simulink model "Squelette_DSPB_ModulateurOQPSK"  (R2016a)
settings: Solver=FixedStepDiscrete  StartTime=0.0  StopTime=1e-3  RelTol=1e-3
InitFcn:
  | %% DSPBuilder Start
  | alt_dspbuilder_update_model(bdroot)
  | %% DSPBuilder End
libraries: allblocks_alteradspbuilder2 x243
(part 2 of 2)

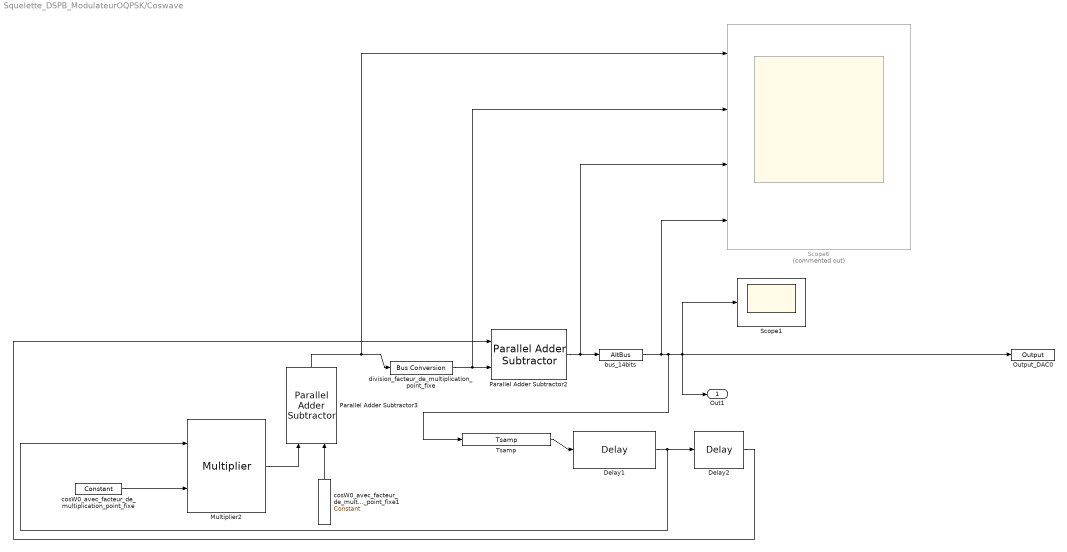
== system Squelette_DSPB_ModulateurOQPSK/Coswave ==
  Delay1 : allblocks_alteradspbuilder2/Delay  pipeline=1  pipeline_display=1  ClockPhase=1  use_ena=off  use_sclr=off  allowFloatingPointOverride=on  logOutputs=off  logFile=U:\S6\Projet\Squelette_ModulateurOQPSK__ORIG\tb_Squelette_DSPB_ModulateurOQPSK\Squelette%5FDSPB%5FModulateurOQPSK_Coswave_Delay1.fixedpointlog  use_init=on  reset_value=0.782390810576588
  Delay2 : allblocks_alteradspbuilder2/Delay  pipeline=1  pipeline_display=1  ClockPhase=1  use_ena=off  use_sclr=off  allowFloatingPointOverride=on  logOutputs=off  logFile=U:\S6\Projet\Squelette_ModulateurOQPSK__ORIG\tb_Squelette_DSPB_ModulateurOQPSK\Squelette%5FDSPB%5FModulateurOQPSK_Coswave_Delay2.fixedpointlog  use_init=on  reset_value=0.224270760949381
  Multiplier2 : allblocks_alteradspbuilder2/Multiplier  BusType=Signed Fractional  bwl=8  bwr=20  pipeline=0  pipeline_display=0  allowFloatingPointOverride=on  logOutputs=off  logFile=U:\S6\Projet\Squelette_ModulateurOQPSK__ORIG\tb_Squelette_DSPB_ModulateurOQPSK\Squelette%5FDSPB%5FModulateurOQPSK_Coswave_Multiplier2.fixedpointlog  UseEqualInputWidth=off  bbwl=8  bbwr=20  FullResolution=on  OutputMsb=8  OutputLsb=0  OutputBwl=16  OutputBwr=16  UseDedicatedCircuitry=YES  use_ena=off  use_aclr=off
  Output_DAC0 : allblocks_alteradspbuilder2/Output  iofile=U:\S6\Projet\Squelette_ModulateurOQPSK__ORIG\tb_Squelette_DSPB_ModulateurOQPSK\Squelette%5FDSPB%5FModulateurOQPSK_Coswave_Output%5FDAC0.capture  BusType=Signed Integer  bwl=14  bwr=0  externalType=Inferred  PORTTYPE=Output  allowFloatingPointOverride=on  logOutputs=off
  Parallel Adder Subtractor2 : allblocks_alteradspbuilder2/Parallel Adder Subtractor  number_of_inputs=2  direction=-+  use_pipeline=off  pipeline_display=0  phase_selection=1  use_ena=off  use_aclr=off  allowFloatingPointOverride=on  logOutputs=off  logFile=U:\S6\Projet\Squelette_ModulateurOQPSK__ORIG\tb_Squelette_DSPB_ModulateurOQPSK\Squelette%5FDSPB%5FModulateurOQPSK_Coswave_Parallel+Adder+Subtractor2.fixedpointlog
  Parallel Adder Subtractor3 : allblocks_alteradspbuilder2/Parallel Adder Subtractor  number_of_inputs=2  direction=+  use_pipeline=off  pipeline_display=0  phase_selection=1  use_ena=off  use_aclr=off  allowFloatingPointOverride=on  logOutputs=off  logFile=U:\S6\Projet\Squelette_ModulateurOQPSK__ORIG\tb_Squelette_DSPB_ModulateurOQPSK\Squelette%5FDSPB%5FModulateurOQPSK_Coswave_Parallel+Adder+Subtractor3.fixedpointlog
  Scope1 : Scope
  Scope6 : Scope  Commented=on  NumInputPorts=4
  Tsamp : allblocks_alteradspbuilder2/Tsamp  SpecifyClock=on  clock=Clock_100MHz
  bus_14bits : allblocks_alteradspbuilder2/AltBus  BusType=Signed Fractional  bwl=14  bwr=14  saturate=off  floatingPointInput=on  floatingPointOutput=on  logOutputs=off  logFile=U:\S6\Projet\Squelette_ModulateurOQPSK__ORIG\tb_Squelette_DSPB_ModulateurOQPSK\Squelette%5FDSPB%5FModulateurOQPSK_Coswave_bus%5F14bits.fixedpointlog
  cosW0_avec_facteur_de_multiplication_point_fixe : allblocks_alteradspbuilder2/Constant  mask_cst=1.564781621153176  BusType=Signed Fractional  bwl=19  bwr=19  roundMode=Truncate  satMode=Wrap  SpecifyClock=off  allowFloatingPointOverride=on  logOutputs=off  logFile=U:\S6\Projet\Squelette_ModulateurOQPSK__ORIG\tb_Squelette_DSPB_ModulateurOQPSK\Squelette%5FDSPB%5FModulateurOQPSK_Coswave_cosW0%5Favec%5Ffacteur%5Fde%5Fmultiplication%5Fpoint%5Ffixe.fixedpointlog
  cosW0_avec_facteur_de_multiplication_point_fixe1 : allblocks_alteradspbuilder2/Constant  mask_cst=2^-15  BusType=Signed Fractional  bwl=8  bwr=40  roundMode=Truncate  satMode=Wrap  SpecifyClock=off  allowFloatingPointOverride=on  logOutputs=off  logFile=U:\S6\Projet\Squelette_ModulateurOQPSK__ORIG\tb_Squelette_DSPB_ModulateurOQPSK\Squelette%5FDSPB%5FModulateurOQPSK_Coswave_cosW0%5Favec%5Ffacteur%5Fde%5Fmultiplication%5Fpoint%5Ffixe1.fixedpointlog
  division_facteur_de_multiplication_point_fixe : allblocks_alteradspbuilder2/Bus Conversion  BusType=Signed Fractional  ibwl=16  ibwr=40  bwl=8  bwr=20  bitToConnectToOutputLSB=16  round=off  saturate=off  pipeline_display=0
  Out1 : Outport
  wires:
  Parallel Adder Subtractor2/1 -> Scope6/3, bus_14bits/1
  Tsamp/1 -> Delay1/1
  cosW0_avec_facteur_de_multiplication_point_fixe1/1 -> Parallel Adder Subtractor3/2
  Multiplier2/1 -> Parallel Adder Subtractor3/1
  division_facteur_de_multiplication_point_fixe/1 -> Scope6/2, Parallel Adder Subtractor2/2
  Delay2/1 -> Parallel Adder Subtractor2/1
  Parallel Adder Subtractor3/1 -> Scope6/1, division_facteur_de_multiplication_point_fixe/1
  Delay1/1 -> Delay2/1, Multiplier2/1
  cosW0_avec_facteur_de_multiplication_point_fixe/1 -> Multiplier2/2
  bus_14bits/1 -> Scope6/4, Out1/1, Scope1/1, Output_DAC0/1, Tsamp/1

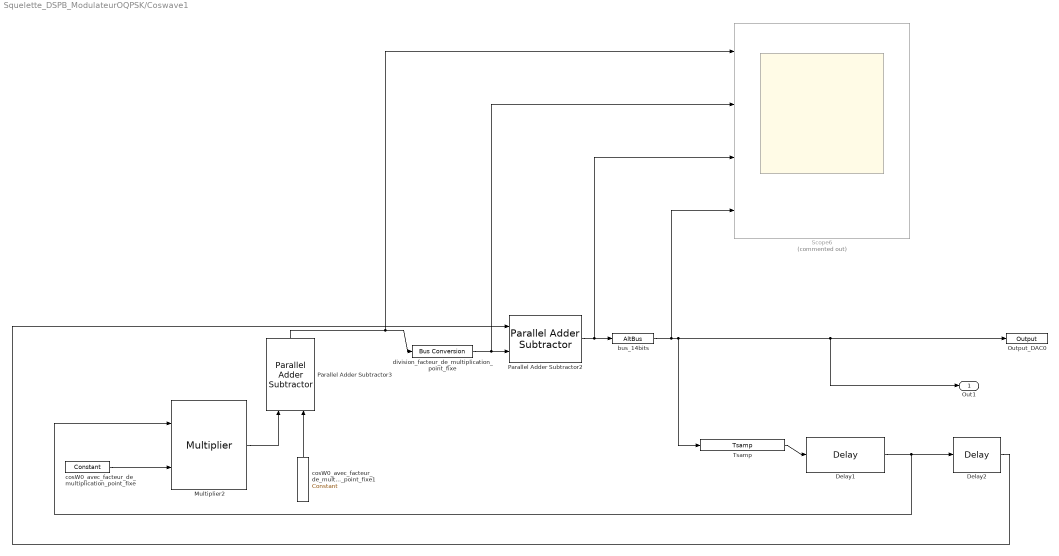
== system Squelette_DSPB_ModulateurOQPSK/Coswave1 ==
  Delay1 : allblocks_alteradspbuilder2/Delay  pipeline=1  pipeline_display=1  ClockPhase=1  use_ena=off  use_sclr=off  allowFloatingPointOverride=on  logOutputs=off  logFile=U:\S6\Projet\Squelette_ModulateurOQPSK__ORIG\tb_Squelette_DSPB_ModulateurOQPSK\Squelette%5FDSPB%5FModulateurOQPSK_Coswave1_Delay1.fixedpointlog  use_init=on  reset_value=0.782390810576588
  Delay2 : allblocks_alteradspbuilder2/Delay  pipeline=1  pipeline_display=1  ClockPhase=1  use_ena=off  use_sclr=off  allowFloatingPointOverride=on  logOutputs=off  logFile=U:\S6\Projet\Squelette_ModulateurOQPSK__ORIG\tb_Squelette_DSPB_ModulateurOQPSK\Squelette%5FDSPB%5FModulateurOQPSK_Coswave1_Delay2.fixedpointlog  use_init=on  reset_value=0.224270760949381
  Multiplier2 : allblocks_alteradspbuilder2/Multiplier  BusType=Signed Fractional  bwl=8  bwr=20  pipeline=0  pipeline_display=0  allowFloatingPointOverride=on  logOutputs=off  logFile=U:\S6\Projet\Squelette_ModulateurOQPSK__ORIG\tb_Squelette_DSPB_ModulateurOQPSK\Squelette%5FDSPB%5FModulateurOQPSK_Coswave1_Multiplier2.fixedpointlog  UseEqualInputWidth=off  bbwl=8  bbwr=20  FullResolution=on  OutputMsb=8  OutputLsb=0  OutputBwl=16  OutputBwr=16  UseDedicatedCircuitry=YES  use_ena=off  use_aclr=off
  Output_DAC0 : allblocks_alteradspbuilder2/Output  iofile=U:\S6\Projet\Squelette_ModulateurOQPSK__ORIG\tb_Squelette_DSPB_ModulateurOQPSK\Squelette%5FDSPB%5FModulateurOQPSK_Coswave1_Output%5FDAC0.capture  BusType=Signed Integer  bwl=14  bwr=0  externalType=Inferred  PORTTYPE=Output  allowFloatingPointOverride=on  logOutputs=off
  Parallel Adder Subtractor2 : allblocks_alteradspbuilder2/Parallel Adder Subtractor  number_of_inputs=2  direction=-+  use_pipeline=off  pipeline_display=0  phase_selection=1  use_ena=off  use_aclr=off  allowFloatingPointOverride=on  logOutputs=off  logFile=U:\S6\Projet\Squelette_ModulateurOQPSK__ORIG\tb_Squelette_DSPB_ModulateurOQPSK\Squelette%5FDSPB%5FModulateurOQPSK_Coswave1_Parallel+Adder+Subtractor2.fixedpointlog
  Parallel Adder Subtractor3 : allblocks_alteradspbuilder2/Parallel Adder Subtractor  number_of_inputs=2  direction=+  use_pipeline=off  pipeline_display=0  phase_selection=1  use_ena=off  use_aclr=off  allowFloatingPointOverride=on  logOutputs=off  logFile=U:\S6\Projet\Squelette_ModulateurOQPSK__ORIG\tb_Squelette_DSPB_ModulateurOQPSK\Squelette%5FDSPB%5FModulateurOQPSK_Coswave1_Parallel+Adder+Subtractor3.fixedpointlog
  Scope6 : Scope  Commented=on  NumInputPorts=4
  Tsamp : allblocks_alteradspbuilder2/Tsamp  SpecifyClock=on  clock=Clock_100MHz
  bus_14bits : allblocks_alteradspbuilder2/AltBus  BusType=Signed Fractional  bwl=14  bwr=14  saturate=off  floatingPointInput=on  floatingPointOutput=on  logOutputs=off  logFile=U:\S6\Projet\Squelette_ModulateurOQPSK__ORIG\tb_Squelette_DSPB_ModulateurOQPSK\Squelette%5FDSPB%5FModulateurOQPSK_Coswave1_bus%5F14bits.fixedpointlog
  cosW0_avec_facteur_de_multiplication_point_fixe : allblocks_alteradspbuilder2/Constant  mask_cst=1.564781621153176  BusType=Signed Fractional  bwl=19  bwr=19  roundMode=Truncate  satMode=Wrap  SpecifyClock=off  allowFloatingPointOverride=on  logOutputs=off  logFile=U:\S6\Projet\Squelette_ModulateurOQPSK__ORIG\tb_Squelette_DSPB_ModulateurOQPSK\Squelette%5FDSPB%5FModulateurOQPSK_Coswave1_cosW0%5Favec%5Ffacteur%5Fde%5Fmultiplication%5Fpoint%5Ffixe.fixedpointlog
  cosW0_avec_facteur_de_multiplication_point_fixe1 : allblocks_alteradspbuilder2/Constant  mask_cst=2^-15  BusType=Signed Fractional  bwl=8  bwr=40  roundMode=Truncate  satMode=Wrap  SpecifyClock=off  allowFloatingPointOverride=on  logOutputs=off  logFile=U:\S6\Projet\Squelette_ModulateurOQPSK__ORIG\tb_Squelette_DSPB_ModulateurOQPSK\Squelette%5FDSPB%5FModulateurOQPSK_Coswave1_cosW0%5Favec%5Ffacteur%5Fde%5Fmultiplication%5Fpoint%5Ffixe1.fixedpointlog
  division_facteur_de_multiplication_point_fixe : allblocks_alteradspbuilder2/Bus Conversion  BusType=Signed Fractional  ibwl=16  ibwr=40  bwl=8  bwr=20  bitToConnectToOutputLSB=16  round=off  saturate=off  pipeline_display=0
  Out1 : Outport
  wires:
  Parallel Adder Subtractor2/1 -> Scope6/3, bus_14bits/1
  Tsamp/1 -> Delay1/1
  cosW0_avec_facteur_de_multiplication_point_fixe1/1 -> Parallel Adder Subtractor3/2
  Multiplier2/1 -> Parallel Adder Subtractor3/1
  division_facteur_de_multiplication_point_fixe/1 -> Scope6/2, Parallel Adder Subtractor2/2
  Delay2/1 -> Parallel Adder Subtractor2/1
  Parallel Adder Subtractor3/1 -> Scope6/1, division_facteur_de_multiplication_point_fixe/1
  Delay1/1 -> Multiplier2/1, Delay2/1
  cosW0_avec_facteur_de_multiplication_point_fixe/1 -> Multiplier2/2
  bus_14bits/1 -> Scope6/4, Out1/1, Output_DAC0/1, Tsamp/1

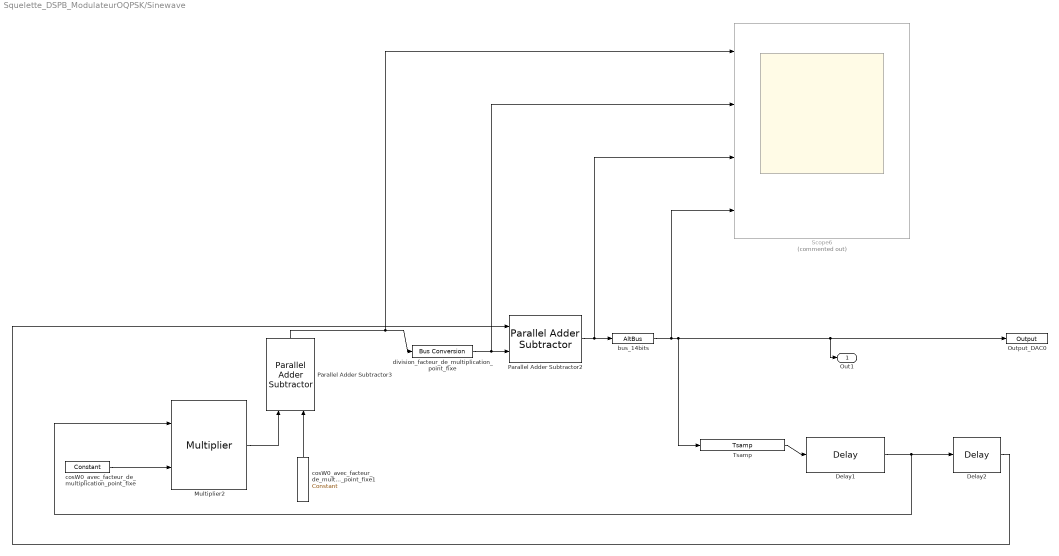
== system Squelette_DSPB_ModulateurOQPSK/Sinewave ==
  Delay1 : allblocks_alteradspbuilder2/Delay  pipeline=1  pipeline_display=1  ClockPhase=1  use_ena=off  use_sclr=off  allowFloatingPointOverride=on  logOutputs=off  logFile=U:\S6\Projet\Squelette_ModulateurOQPSK__ORIG\tb_Squelette_DSPB_ModulateurOQPSK\Squelette%5FDSPB%5FModulateurOQPSK_Sinewave_Delay1.fixedpointlog  use_init=on  reset_value=0.622787780488113
  Delay2 : allblocks_alteradspbuilder2/Delay  pipeline=1  pipeline_display=1  ClockPhase=1  use_ena=off  use_sclr=off  allowFloatingPointOverride=on  logOutputs=off  logFile=U:\S6\Projet\Squelette_ModulateurOQPSK__ORIG\tb_Squelette_DSPB_ModulateurOQPSK\Squelette%5FDSPB%5FModulateurOQPSK_Sinewave_Delay2.fixedpointlog  use_init=on  reset_value=0.974526872786577
  Multiplier2 : allblocks_alteradspbuilder2/Multiplier  BusType=Signed Fractional  bwl=8  bwr=20  pipeline=0  pipeline_display=0  allowFloatingPointOverride=on  logOutputs=off  logFile=U:\S6\Projet\Squelette_ModulateurOQPSK__ORIG\tb_Squelette_DSPB_ModulateurOQPSK\Squelette%5FDSPB%5FModulateurOQPSK_Sinewave_Multiplier2.fixedpointlog  UseEqualInputWidth=off  bbwl=8  bbwr=20  FullResolution=on  OutputMsb=8  OutputLsb=0  OutputBwl=16  OutputBwr=16  UseDedicatedCircuitry=YES  use_ena=off  use_aclr=off
  Output_DAC0 : allblocks_alteradspbuilder2/Output  iofile=U:\S6\Projet\Squelette_ModulateurOQPSK__ORIG\tb_Squelette_DSPB_ModulateurOQPSK\Squelette%5FDSPB%5FModulateurOQPSK_Sinewave_Output%5FDAC0.capture  BusType=Signed Integer  bwl=14  bwr=0  externalType=Inferred  PORTTYPE=Output  allowFloatingPointOverride=on  logOutputs=off
  Parallel Adder Subtractor2 : allblocks_alteradspbuilder2/Parallel Adder Subtractor  number_of_inputs=2  direction=-+  use_pipeline=off  pipeline_display=0  phase_selection=1  use_ena=off  use_aclr=off  allowFloatingPointOverride=on  logOutputs=off  logFile=U:\S6\Projet\Squelette_ModulateurOQPSK__ORIG\tb_Squelette_DSPB_ModulateurOQPSK\Squelette%5FDSPB%5FModulateurOQPSK_Sinewave_Parallel+Adder+Subtractor2.fixedpointlog
  Parallel Adder Subtractor3 : allblocks_alteradspbuilder2/Parallel Adder Subtractor  number_of_inputs=2  direction=+  use_pipeline=off  pipeline_display=0  phase_selection=1  use_ena=off  use_aclr=off  allowFloatingPointOverride=on  logOutputs=off  logFile=U:\S6\Projet\Squelette_ModulateurOQPSK__ORIG\tb_Squelette_DSPB_ModulateurOQPSK\Squelette%5FDSPB%5FModulateurOQPSK_Sinewave_Parallel+Adder+Subtractor3.fixedpointlog
  Scope6 : Scope  Commented=on  NumInputPorts=4
  Tsamp : allblocks_alteradspbuilder2/Tsamp  SpecifyClock=on  clock=Clock_100MHz
  bus_14bits : allblocks_alteradspbuilder2/AltBus  BusType=Signed Fractional  bwl=14  bwr=14  saturate=off  floatingPointInput=on  floatingPointOutput=on  logOutputs=off  logFile=U:\S6\Projet\Squelette_ModulateurOQPSK__ORIG\tb_Squelette_DSPB_ModulateurOQPSK\Squelette%5FDSPB%5FModulateurOQPSK_Sinewave_bus%5F14bits.fixedpointlog
  cosW0_avec_facteur_de_multiplication_point_fixe : allblocks_alteradspbuilder2/Constant  mask_cst=1.564781621153176  BusType=Signed Fractional  bwl=19  bwr=19  roundMode=Truncate  satMode=Wrap  SpecifyClock=off  allowFloatingPointOverride=on  logOutputs=off  logFile=U:\S6\Projet\Squelette_ModulateurOQPSK__ORIG\tb_Squelette_DSPB_ModulateurOQPSK\Squelette%5FDSPB%5FModulateurOQPSK_Sinewave_cosW0%5Favec%5Ffacteur%5Fde%5Fmultiplication%5Fpoint%5Ffixe.fixedpointlog
  cosW0_avec_facteur_de_multiplication_point_fixe1 : allblocks_alteradspbuilder2/Constant  mask_cst=2^-15  BusType=Signed Fractional  bwl=8  bwr=40  roundMode=Truncate  satMode=Wrap  SpecifyClock=off  allowFloatingPointOverride=on  logOutputs=off  logFile=U:\S6\Projet\Squelette_ModulateurOQPSK__ORIG\tb_Squelette_DSPB_ModulateurOQPSK\Squelette%5FDSPB%5FModulateurOQPSK_Sinewave_cosW0%5Favec%5Ffacteur%5Fde%5Fmultiplication%5Fpoint%5Ffixe1.fixedpointlog
  division_facteur_de_multiplication_point_fixe : allblocks_alteradspbuilder2/Bus Conversion  BusType=Signed Fractional  ibwl=16  ibwr=40  bwl=8  bwr=20  bitToConnectToOutputLSB=16  round=off  saturate=off  pipeline_display=0
  Out1 : Outport
  wires:
  Parallel Adder Subtractor2/1 -> Scope6/3, bus_14bits/1
  Tsamp/1 -> Delay1/1
  cosW0_avec_facteur_de_multiplication_point_fixe1/1 -> Parallel Adder Subtractor3/2
  Multiplier2/1 -> Parallel Adder Subtractor3/1
  division_facteur_de_multiplication_point_fixe/1 -> Scope6/2, Parallel Adder Subtractor2/2
  Delay2/1 -> Parallel Adder Subtractor2/1
  Parallel Adder Subtractor3/1 -> Scope6/1, division_facteur_de_multiplication_point_fixe/1
  Delay1/1 -> Multiplier2/1, Delay2/1
  cosW0_avec_facteur_de_multiplication_point_fixe/1 -> Multiplier2/2
  bus_14bits/1 -> Scope6/4, Out1/1, Output_DAC0/1, Tsamp/1

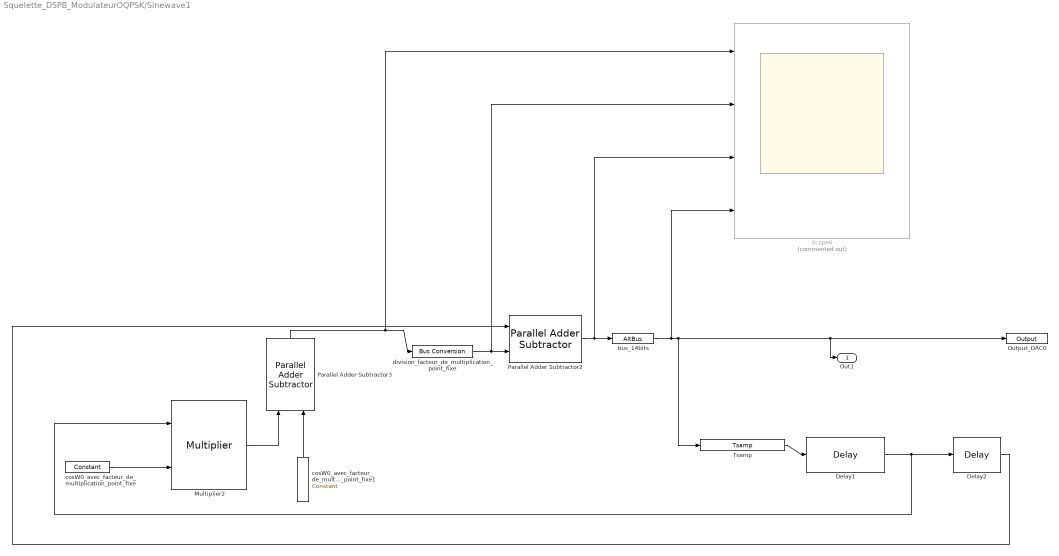
== system Squelette_DSPB_ModulateurOQPSK/Sinewave1 ==
  Delay1 : allblocks_alteradspbuilder2/Delay  pipeline=1  pipeline_display=1  ClockPhase=1  use_ena=off  use_sclr=off  allowFloatingPointOverride=on  logOutputs=off  logFile=U:\S6\Projet\Squelette_ModulateurOQPSK__ORIG\tb_Squelette_DSPB_ModulateurOQPSK\Squelette%5FDSPB%5FModulateurOQPSK_Sinewave1_Delay1.fixedpointlog  use_init=on  reset_value=0.031410759078128
  Delay2 : allblocks_alteradspbuilder2/Delay  pipeline=1  pipeline_display=1  ClockPhase=1  use_ena=off  use_sclr=off  allowFloatingPointOverride=on  logOutputs=off  logFile=U:\S6\Projet\Squelette_ModulateurOQPSK__ORIG\tb_Squelette_DSPB_ModulateurOQPSK\Squelette%5FDSPB%5FModulateurOQPSK_Sinewave1_Delay2.fixedpointlog  use_init=on  reset_value=0.062790519529314
  Multiplier2 : allblocks_alteradspbuilder2/Multiplier  BusType=Signed Fractional  bwl=8  bwr=20  pipeline=0  pipeline_display=0  allowFloatingPointOverride=on  logOutputs=off  logFile=U:\S6\Projet\Squelette_ModulateurOQPSK__ORIG\tb_Squelette_DSPB_ModulateurOQPSK\Squelette%5FDSPB%5FModulateurOQPSK_Sinewave1_Multiplier2.fixedpointlog  UseEqualInputWidth=off  bbwl=8  bbwr=20  FullResolution=on  OutputMsb=8  OutputLsb=0  OutputBwl=16  OutputBwr=16  UseDedicatedCircuitry=YES  use_ena=off  use_aclr=off
  Output_DAC0 : allblocks_alteradspbuilder2/Output  iofile=U:\S6\Projet\Squelette_ModulateurOQPSK__ORIG\tb_Squelette_DSPB_ModulateurOQPSK\Squelette%5FDSPB%5FModulateurOQPSK_Sinewave1_Output%5FDAC0.capture  BusType=Signed Integer  bwl=14  bwr=0  externalType=Inferred  PORTTYPE=Output  allowFloatingPointOverride=on  logOutputs=off
  Parallel Adder Subtractor2 : allblocks_alteradspbuilder2/Parallel Adder Subtractor  number_of_inputs=2  direction=-+  use_pipeline=off  pipeline_display=0  phase_selection=1  use_ena=off  use_aclr=off  allowFloatingPointOverride=on  logOutputs=off  logFile=U:\S6\Projet\Squelette_ModulateurOQPSK__ORIG\tb_Squelette_DSPB_ModulateurOQPSK\Squelette%5FDSPB%5FModulateurOQPSK_Sinewave1_Parallel+Adder+Subtractor2.fixedpointlog
  Parallel Adder Subtractor3 : allblocks_alteradspbuilder2/Parallel Adder Subtractor  number_of_inputs=2  direction=+  use_pipeline=off  pipeline_display=0  phase_selection=1  use_ena=off  use_aclr=off  allowFloatingPointOverride=on  logOutputs=off  logFile=U:\S6\Projet\Squelette_ModulateurOQPSK__ORIG\tb_Squelette_DSPB_ModulateurOQPSK\Squelette%5FDSPB%5FModulateurOQPSK_Sinewave1_Parallel+Adder+Subtractor3.fixedpointlog
  Scope6 : Scope  Commented=on  NumInputPorts=4
  Tsamp : allblocks_alteradspbuilder2/Tsamp  SpecifyClock=on  clock=Clock_100MHz
  bus_14bits : allblocks_alteradspbuilder2/AltBus  BusType=Signed Fractional  bwl=14  bwr=14  saturate=off  floatingPointInput=on  floatingPointOutput=on  logOutputs=off  logFile=U:\S6\Projet\Squelette_ModulateurOQPSK__ORIG\tb_Squelette_DSPB_ModulateurOQPSK\Squelette%5FDSPB%5FModulateurOQPSK_Sinewave1_bus%5F14bits.fixedpointlog
  cosW0_avec_facteur_de_multiplication_point_fixe : allblocks_alteradspbuilder2/Constant  mask_cst=1.999013120731463  BusType=Signed Fractional  bwl=19  bwr=19  roundMode=Truncate  satMode=Wrap  SpecifyClock=off  allowFloatingPointOverride=on  logOutputs=off  logFile=U:\S6\Projet\Squelette_ModulateurOQPSK__ORIG\tb_Squelette_DSPB_ModulateurOQPSK\Squelette%5FDSPB%5FModulateurOQPSK_Sinewave1_cosW0%5Favec%5Ffacteur%5Fde%5Fmultiplication%5Fpoint%5Ffixe.fixedpointlog
  cosW0_avec_facteur_de_multiplication_point_fixe1 : allblocks_alteradspbuilder2/Constant  mask_cst=2^-15  BusType=Signed Fractional  bwl=8  bwr=40  roundMode=Truncate  satMode=Wrap  SpecifyClock=off  allowFloatingPointOverride=on  logOutputs=off  logFile=U:\S6\Projet\Squelette_ModulateurOQPSK__ORIG\tb_Squelette_DSPB_ModulateurOQPSK\Squelette%5FDSPB%5FModulateurOQPSK_Sinewave1_cosW0%5Favec%5Ffacteur%5Fde%5Fmultiplication%5Fpoint%5Ffixe1.fixedpointlog
  division_facteur_de_multiplication_point_fixe : allblocks_alteradspbuilder2/Bus Conversion  BusType=Signed Fractional  ibwl=16  ibwr=40  bwl=8  bwr=20  bitToConnectToOutputLSB=16  round=off  saturate=off  pipeline_display=0
  Out1 : Outport
  wires:
  Parallel Adder Subtractor2/1 -> Scope6/3, bus_14bits/1
  Tsamp/1 -> Delay1/1
  cosW0_avec_facteur_de_multiplication_point_fixe1/1 -> Parallel Adder Subtractor3/2
  Multiplier2/1 -> Parallel Adder Subtractor3/1
  division_facteur_de_multiplication_point_fixe/1 -> Scope6/2, Parallel Adder Subtractor2/2
  Delay2/1 -> Parallel Adder Subtractor2/1
  Parallel Adder Subtractor3/1 -> Scope6/1, division_facteur_de_multiplication_point_fixe/1
  Delay1/1 -> Multiplier2/1, Delay2/1
  cosW0_avec_facteur_de_multiplication_point_fixe/1 -> Multiplier2/2
  bus_14bits/1 -> Scope6/4, Out1/1, Output_DAC0/1, Tsamp/1

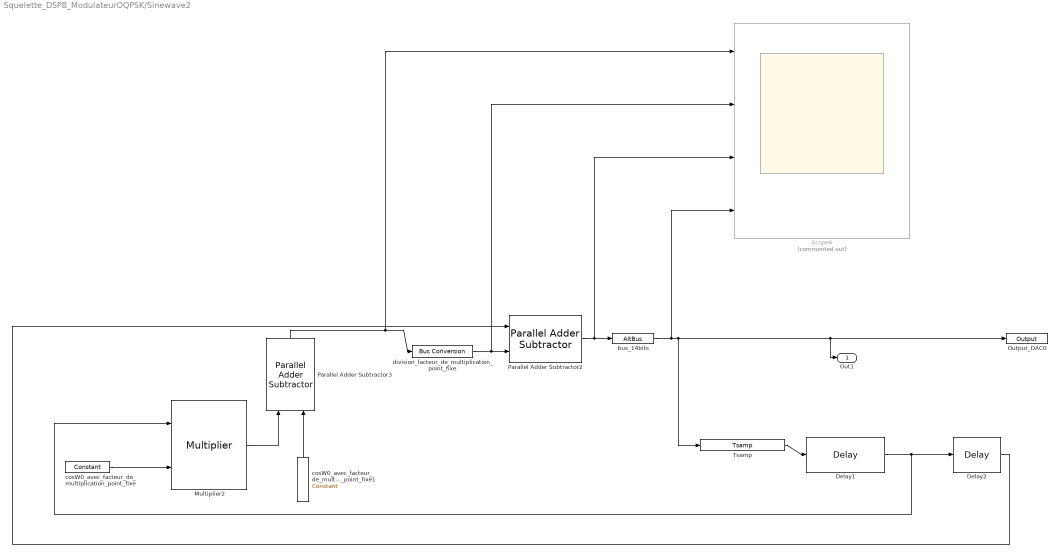
== system Squelette_DSPB_ModulateurOQPSK/Sinewave2 ==
  Delay1 : allblocks_alteradspbuilder2/Delay  pipeline=1  pipeline_display=1  ClockPhase=1  use_ena=off  use_sclr=off  allowFloatingPointOverride=on  logOutputs=off  logFile=U:\S6\Projet\Squelette_ModulateurOQPSK__ORIG\tb_Squelette_DSPB_ModulateurOQPSK\Squelette%5FDSPB%5FModulateurOQPSK_Sinewave2_Delay1.fixedpointlog  use_init=on  reset_value=0.031410759078128
  Delay2 : allblocks_alteradspbuilder2/Delay  pipeline=1  pipeline_display=1  ClockPhase=1  use_ena=off  use_sclr=off  allowFloatingPointOverride=on  logOutputs=off  logFile=U:\S6\Projet\Squelette_ModulateurOQPSK__ORIG\tb_Squelette_DSPB_ModulateurOQPSK\Squelette%5FDSPB%5FModulateurOQPSK_Sinewave2_Delay2.fixedpointlog  use_init=on  reset_value=0.062790519529314
  Multiplier2 : allblocks_alteradspbuilder2/Multiplier  BusType=Signed Fractional  bwl=8  bwr=20  pipeline=0  pipeline_display=0  allowFloatingPointOverride=on  logOutputs=off  logFile=U:\S6\Projet\Squelette_ModulateurOQPSK__ORIG\tb_Squelette_DSPB_ModulateurOQPSK\Squelette%5FDSPB%5FModulateurOQPSK_Sinewave2_Multiplier2.fixedpointlog  UseEqualInputWidth=off  bbwl=8  bbwr=20  FullResolution=on  OutputMsb=8  OutputLsb=0  OutputBwl=16  OutputBwr=16  UseDedicatedCircuitry=YES  use_ena=off  use_aclr=off
  Output_DAC0 : allblocks_alteradspbuilder2/Output  iofile=U:\S6\Projet\Squelette_ModulateurOQPSK__ORIG\tb_Squelette_DSPB_ModulateurOQPSK\Squelette%5FDSPB%5FModulateurOQPSK_Sinewave2_Output%5FDAC0.capture  BusType=Signed Integer  bwl=14  bwr=0  externalType=Inferred  PORTTYPE=Output  allowFloatingPointOverride=on  logOutputs=off
  Parallel Adder Subtractor2 : allblocks_alteradspbuilder2/Parallel Adder Subtractor  number_of_inputs=2  direction=-+  use_pipeline=off  pipeline_display=0  phase_selection=1  use_ena=off  use_aclr=off  allowFloatingPointOverride=on  logOutputs=off  logFile=U:\S6\Projet\Squelette_ModulateurOQPSK__ORIG\tb_Squelette_DSPB_ModulateurOQPSK\Squelette%5FDSPB%5FModulateurOQPSK_Sinewave2_Parallel+Adder+Subtractor2.fixedpointlog
  Parallel Adder Subtractor3 : allblocks_alteradspbuilder2/Parallel Adder Subtractor  number_of_inputs=2  direction=+  use_pipeline=off  pipeline_display=0  phase_selection=1  use_ena=off  use_aclr=off  allowFloatingPointOverride=on  logOutputs=off  logFile=U:\S6\Projet\Squelette_ModulateurOQPSK__ORIG\tb_Squelette_DSPB_ModulateurOQPSK\Squelette%5FDSPB%5FModulateurOQPSK_Sinewave2_Parallel+Adder+Subtractor3.fixedpointlog
  Scope6 : Scope  Commented=on  NumInputPorts=4
  Tsamp : allblocks_alteradspbuilder2/Tsamp  SpecifyClock=on  clock=Clock_100MHz
  bus_14bits : allblocks_alteradspbuilder2/AltBus  BusType=Signed Fractional  bwl=14  bwr=14  saturate=off  floatingPointInput=on  floatingPointOutput=on  logOutputs=off  logFile=U:\S6\Projet\Squelette_ModulateurOQPSK__ORIG\tb_Squelette_DSPB_ModulateurOQPSK\Squelette%5FDSPB%5FModulateurOQPSK_Sinewave2_bus%5F14bits.fixedpointlog
  cosW0_avec_facteur_de_multiplication_point_fixe : allblocks_alteradspbuilder2/Constant  mask_cst=1.999013120731463  BusType=Signed Fractional  bwl=19  bwr=19  roundMode=Truncate  satMode=Wrap  SpecifyClock=off  allowFloatingPointOverride=on  logOutputs=off  logFile=U:\S6\Projet\Squelette_ModulateurOQPSK__ORIG\tb_Squelette_DSPB_ModulateurOQPSK\Squelette%5FDSPB%5FModulateurOQPSK_Sinewave2_cosW0%5Favec%5Ffacteur%5Fde%5Fmultiplication%5Fpoint%5Ffixe.fixedpointlog
  cosW0_avec_facteur_de_multiplication_point_fixe1 : allblocks_alteradspbuilder2/Constant  mask_cst=2^-15  BusType=Signed Fractional  bwl=8  bwr=40  roundMode=Truncate  satMode=Wrap  SpecifyClock=off  allowFloatingPointOverride=on  logOutputs=off  logFile=U:\S6\Projet\Squelette_ModulateurOQPSK__ORIG\tb_Squelette_DSPB_ModulateurOQPSK\Squelette%5FDSPB%5FModulateurOQPSK_Sinewave2_cosW0%5Favec%5Ffacteur%5Fde%5Fmultiplication%5Fpoint%5Ffixe1.fixedpointlog
  division_facteur_de_multiplication_point_fixe : allblocks_alteradspbuilder2/Bus Conversion  BusType=Signed Fractional  ibwl=16  ibwr=40  bwl=8  bwr=20  bitToConnectToOutputLSB=16  round=off  saturate=off  pipeline_display=0
  Out1 : Outport
  wires:
  Parallel Adder Subtractor2/1 -> Scope6/3, bus_14bits/1
  Tsamp/1 -> Delay1/1
  cosW0_avec_facteur_de_multiplication_point_fixe1/1 -> Parallel Adder Subtractor3/2
  Multiplier2/1 -> Parallel Adder Subtractor3/1
  division_facteur_de_multiplication_point_fixe/1 -> Scope6/2, Parallel Adder Subtractor2/2
  Delay2/1 -> Parallel Adder Subtractor2/1
  Parallel Adder Subtractor3/1 -> Scope6/1, division_facteur_de_multiplication_point_fixe/1
  Delay1/1 -> Multiplier2/1, Delay2/1
  cosW0_avec_facteur_de_multiplication_point_fixe/1 -> Multiplier2/2
  bus_14bits/1 -> Scope6/4, Out1/1, Output_DAC0/1, Tsamp/1

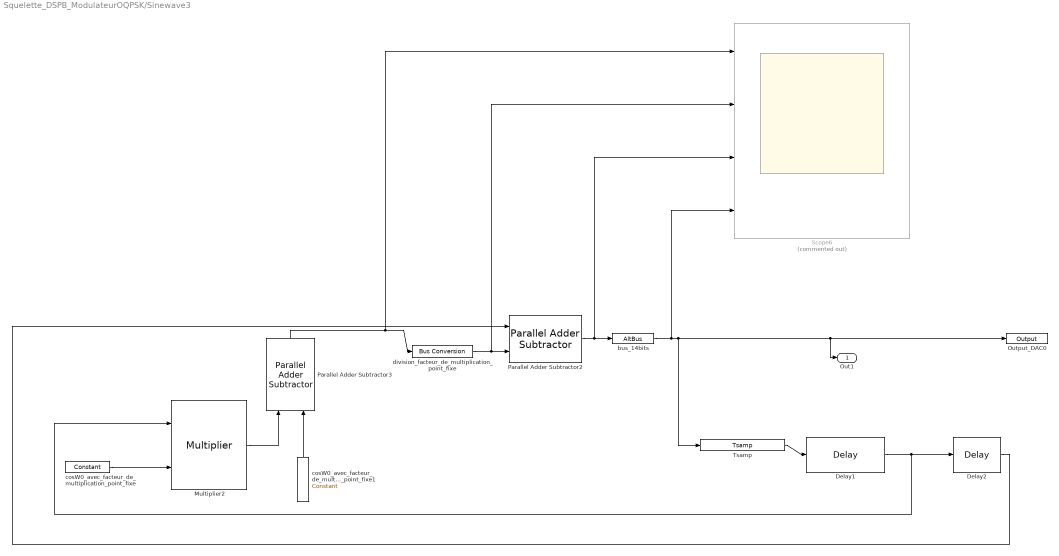
== system Squelette_DSPB_ModulateurOQPSK/Sinewave3 ==
  Delay1 : allblocks_alteradspbuilder2/Delay  pipeline=1  pipeline_display=1  ClockPhase=1  use_ena=off  use_sclr=off  allowFloatingPointOverride=on  logOutputs=off  logFile=U:\S6\Projet\Squelette_ModulateurOQPSK__ORIG\tb_Squelette_DSPB_ModulateurOQPSK\Squelette%5FDSPB%5FModulateurOQPSK_Sinewave3_Delay1.fixedpointlog  use_init=on  reset_value=0.622787780488113
  Delay2 : allblocks_alteradspbuilder2/Delay  pipeline=1  pipeline_display=1  ClockPhase=1  use_ena=off  use_sclr=off  allowFloatingPointOverride=on  logOutputs=off  logFile=U:\S6\Projet\Squelette_ModulateurOQPSK__ORIG\tb_Squelette_DSPB_ModulateurOQPSK\Squelette%5FDSPB%5FModulateurOQPSK_Sinewave3_Delay2.fixedpointlog  use_init=on  reset_value=0.974526872786577
  Multiplier2 : allblocks_alteradspbuilder2/Multiplier  BusType=Signed Fractional  bwl=8  bwr=20  pipeline=0  pipeline_display=0  allowFloatingPointOverride=on  logOutputs=off  logFile=U:\S6\Projet\Squelette_ModulateurOQPSK__ORIG\tb_Squelette_DSPB_ModulateurOQPSK\Squelette%5FDSPB%5FModulateurOQPSK_Sinewave3_Multiplier2.fixedpointlog  UseEqualInputWidth=off  bbwl=8  bbwr=20  FullResolution=on  OutputMsb=8  OutputLsb=0  OutputBwl=16  OutputBwr=16  UseDedicatedCircuitry=YES  use_ena=off  use_aclr=off
  Output_DAC0 : allblocks_alteradspbuilder2/Output  iofile=U:\S6\Projet\Squelette_ModulateurOQPSK__ORIG\tb_Squelette_DSPB_ModulateurOQPSK\Squelette%5FDSPB%5FModulateurOQPSK_Sinewave3_Output%5FDAC0.capture  BusType=Signed Integer  bwl=14  bwr=0  externalType=Inferred  PORTTYPE=Output  allowFloatingPointOverride=on  logOutputs=off
  Parallel Adder Subtractor2 : allblocks_alteradspbuilder2/Parallel Adder Subtractor  number_of_inputs=2  direction=-+  use_pipeline=off  pipeline_display=0  phase_selection=1  use_ena=off  use_aclr=off  allowFloatingPointOverride=on  logOutputs=off  logFile=U:\S6\Projet\Squelette_ModulateurOQPSK__ORIG\tb_Squelette_DSPB_ModulateurOQPSK\Squelette%5FDSPB%5FModulateurOQPSK_Sinewave3_Parallel+Adder+Subtractor2.fixedpointlog
  Parallel Adder Subtractor3 : allblocks_alteradspbuilder2/Parallel Adder Subtractor  number_of_inputs=2  direction=+  use_pipeline=off  pipeline_display=0  phase_selection=1  use_ena=off  use_aclr=off  allowFloatingPointOverride=on  logOutputs=off  logFile=U:\S6\Projet\Squelette_ModulateurOQPSK__ORIG\tb_Squelette_DSPB_ModulateurOQPSK\Squelette%5FDSPB%5FModulateurOQPSK_Sinewave3_Parallel+Adder+Subtractor3.fixedpointlog
  Scope6 : Scope  Commented=on  NumInputPorts=4
  Tsamp : allblocks_alteradspbuilder2/Tsamp  SpecifyClock=on  clock=Clock_100MHz
  bus_14bits : allblocks_alteradspbuilder2/AltBus  BusType=Signed Fractional  bwl=14  bwr=14  saturate=off  floatingPointInput=on  floatingPointOutput=on  logOutputs=off  logFile=U:\S6\Projet\Squelette_ModulateurOQPSK__ORIG\tb_Squelette_DSPB_ModulateurOQPSK\Squelette%5FDSPB%5FModulateurOQPSK_Sinewave3_bus%5F14bits.fixedpointlog
  cosW0_avec_facteur_de_multiplication_point_fixe : allblocks_alteradspbuilder2/Constant  mask_cst=1.564781621153176  BusType=Signed Fractional  bwl=19  bwr=19  roundMode=Truncate  satMode=Wrap  SpecifyClock=off  allowFloatingPointOverride=on  logOutputs=off  logFile=U:\S6\Projet\Squelette_ModulateurOQPSK__ORIG\tb_Squelette_DSPB_ModulateurOQPSK\Squelette%5FDSPB%5FModulateurOQPSK_Sinewave3_cosW0%5Favec%5Ffacteur%5Fde%5Fmultiplication%5Fpoint%5Ffixe.fixedpointlog
  cosW0_avec_facteur_de_multiplication_point_fixe1 : allblocks_alteradspbuilder2/Constant  mask_cst=2^-15  BusType=Signed Fractional  bwl=8  bwr=40  roundMode=Truncate  satMode=Wrap  SpecifyClock=off  allowFloatingPointOverride=on  logOutputs=off  logFile=U:\S6\Projet\Squelette_ModulateurOQPSK__ORIG\tb_Squelette_DSPB_ModulateurOQPSK\Squelette%5FDSPB%5FModulateurOQPSK_Sinewave3_cosW0%5Favec%5Ffacteur%5Fde%5Fmultiplication%5Fpoint%5Ffixe1.fixedpointlog
  division_facteur_de_multiplication_point_fixe : allblocks_alteradspbuilder2/Bus Conversion  BusType=Signed Fractional  ibwl=16  ibwr=40  bwl=8  bwr=20  bitToConnectToOutputLSB=16  round=off  saturate=off  pipeline_display=0
  Out1 : Outport
  wires:
  Parallel Adder Subtractor2/1 -> Scope6/3, bus_14bits/1
  Tsamp/1 -> Delay1/1
  cosW0_avec_facteur_de_multiplication_point_fixe1/1 -> Parallel Adder Subtractor3/2
  Multiplier2/1 -> Parallel Adder Subtractor3/1
  division_facteur_de_multiplication_point_fixe/1 -> Scope6/2, Parallel Adder Subtractor2/2
  Delay2/1 -> Parallel Adder Subtractor2/1
  Parallel Adder Subtractor3/1 -> Scope6/1, division_facteur_de_multiplication_point_fixe/1
  Delay1/1 -> Multiplier2/1, Delay2/1
  cosW0_avec_facteur_de_multiplication_point_fixe/1 -> Multiplier2/2
  bus_14bits/1 -> Scope6/4, Out1/1, Output_DAC0/1, Tsamp/1

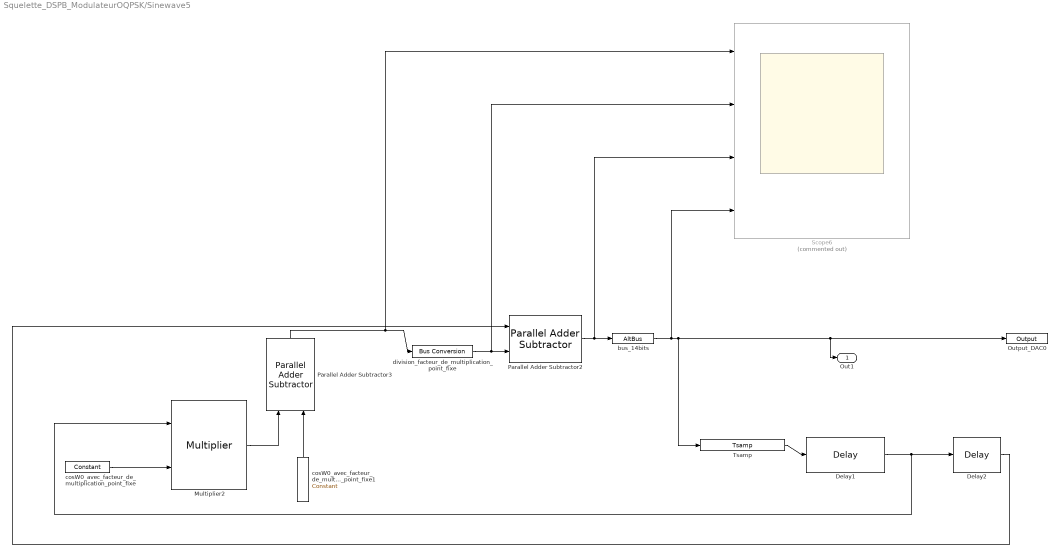
== system Squelette_DSPB_ModulateurOQPSK/Sinewave5 ==
  Delay1 : allblocks_alteradspbuilder2/Delay  pipeline=1  pipeline_display=1  ClockPhase=1  use_ena=off  use_sclr=off  allowFloatingPointOverride=on  logOutputs=off  logFile=U:\S6\Projet\Squelette_ModulateurOQPSK__ORIG\tb_Squelette_DSPB_ModulateurOQPSK\Squelette%5FDSPB%5FModulateurOQPSK_Sinewave5_Delay1.fixedpointlog  use_init=on  reset_value=0.031410759078128
  Delay2 : allblocks_alteradspbuilder2/Delay  pipeline=1  pipeline_display=1  ClockPhase=1  use_ena=off  use_sclr=off  allowFloatingPointOverride=on  logOutputs=off  logFile=U:\S6\Projet\Squelette_ModulateurOQPSK__ORIG\tb_Squelette_DSPB_ModulateurOQPSK\Squelette%5FDSPB%5FModulateurOQPSK_Sinewave5_Delay2.fixedpointlog  use_init=on  reset_value=0.062790519529314
  Multiplier2 : allblocks_alteradspbuilder2/Multiplier  BusType=Signed Fractional  bwl=8  bwr=20  pipeline=0  pipeline_display=0  allowFloatingPointOverride=on  logOutputs=off  logFile=U:\S6\Projet\Squelette_ModulateurOQPSK__ORIG\tb_Squelette_DSPB_ModulateurOQPSK\Squelette%5FDSPB%5FModulateurOQPSK_Sinewave5_Multiplier2.fixedpointlog  UseEqualInputWidth=off  bbwl=8  bbwr=20  FullResolution=on  OutputMsb=8  OutputLsb=0  OutputBwl=16  OutputBwr=16  UseDedicatedCircuitry=YES  use_ena=off  use_aclr=off
  Output_DAC0 : allblocks_alteradspbuilder2/Output  iofile=U:\S6\Projet\Squelette_ModulateurOQPSK__ORIG\tb_Squelette_DSPB_ModulateurOQPSK\Squelette%5FDSPB%5FModulateurOQPSK_Sinewave5_Output%5FDAC0.capture  BusType=Signed Integer  bwl=14  bwr=0  externalType=Inferred  PORTTYPE=Output  allowFloatingPointOverride=on  logOutputs=off
  Parallel Adder Subtractor2 : allblocks_alteradspbuilder2/Parallel Adder Subtractor  number_of_inputs=2  direction=-+  use_pipeline=off  pipeline_display=0  phase_selection=1  use_ena=off  use_aclr=off  allowFloatingPointOverride=on  logOutputs=off  logFile=U:\S6\Projet\Squelette_ModulateurOQPSK__ORIG\tb_Squelette_DSPB_ModulateurOQPSK\Squelette%5FDSPB%5FModulateurOQPSK_Sinewave5_Parallel+Adder+Subtractor2.fixedpointlog
  Parallel Adder Subtractor3 : allblocks_alteradspbuilder2/Parallel Adder Subtractor  number_of_inputs=2  direction=+  use_pipeline=off  pipeline_display=0  phase_selection=1  use_ena=off  use_aclr=off  allowFloatingPointOverride=on  logOutputs=off  logFile=U:\S6\Projet\Squelette_ModulateurOQPSK__ORIG\tb_Squelette_DSPB_ModulateurOQPSK\Squelette%5FDSPB%5FModulateurOQPSK_Sinewave5_Parallel+Adder+Subtractor3.fixedpointlog
  Scope6 : Scope  Commented=on  NumInputPorts=4
  Tsamp : allblocks_alteradspbuilder2/Tsamp  SpecifyClock=on  clock=Clock_100MHz
  bus_14bits : allblocks_alteradspbuilder2/AltBus  BusType=Signed Fractional  bwl=14  bwr=14  saturate=off  floatingPointInput=on  floatingPointOutput=on  logOutputs=off  logFile=U:\S6\Projet\Squelette_ModulateurOQPSK__ORIG\tb_Squelette_DSPB_ModulateurOQPSK\Squelette%5FDSPB%5FModulateurOQPSK_Sinewave5_bus%5F14bits.fixedpointlog
  cosW0_avec_facteur_de_multiplication_point_fixe : allblocks_alteradspbuilder2/Constant  mask_cst=1.999013120731463  BusType=Signed Fractional  bwl=19  bwr=19  roundMode=Truncate  satMode=Wrap  SpecifyClock=off  allowFloatingPointOverride=on  logOutputs=off  logFile=U:\S6\Projet\Squelette_ModulateurOQPSK__ORIG\tb_Squelette_DSPB_ModulateurOQPSK\Squelette%5FDSPB%5FModulateurOQPSK_Sinewave5_cosW0%5Favec%5Ffacteur%5Fde%5Fmultiplication%5Fpoint%5Ffixe.fixedpointlog
  cosW0_avec_facteur_de_multiplication_point_fixe1 : allblocks_alteradspbuilder2/Constant  mask_cst=2^-15  BusType=Signed Fractional  bwl=8  bwr=40  roundMode=Truncate  satMode=Wrap  SpecifyClock=off  allowFloatingPointOverride=on  logOutputs=off  logFile=U:\S6\Projet\Squelette_ModulateurOQPSK__ORIG\tb_Squelette_DSPB_ModulateurOQPSK\Squelette%5FDSPB%5FModulateurOQPSK_Sinewave5_cosW0%5Favec%5Ffacteur%5Fde%5Fmultiplication%5Fpoint%5Ffixe1.fixedpointlog
  division_facteur_de_multiplication_point_fixe : allblocks_alteradspbuilder2/Bus Conversion  BusType=Signed Fractional  ibwl=16  ibwr=40  bwl=8  bwr=20  bitToConnectToOutputLSB=16  round=off  saturate=off  pipeline_display=0
  Out1 : Outport
  wires:
  Parallel Adder Subtractor2/1 -> Scope6/3, bus_14bits/1
  Tsamp/1 -> Delay1/1
  cosW0_avec_facteur_de_multiplication_point_fixe1/1 -> Parallel Adder Subtractor3/2
  Multiplier2/1 -> Parallel Adder Subtractor3/1
  division_facteur_de_multiplication_point_fixe/1 -> Scope6/2, Parallel Adder Subtractor2/2
  Delay2/1 -> Parallel Adder Subtractor2/1
  Parallel Adder Subtractor3/1 -> Scope6/1, division_facteur_de_multiplication_point_fixe/1
  Delay1/1 -> Multiplier2/1, Delay2/1
  cosW0_avec_facteur_de_multiplication_point_fixe/1 -> Multiplier2/2
  bus_14bits/1 -> Scope6/4, Out1/1, Output_DAC0/1, Tsamp/1

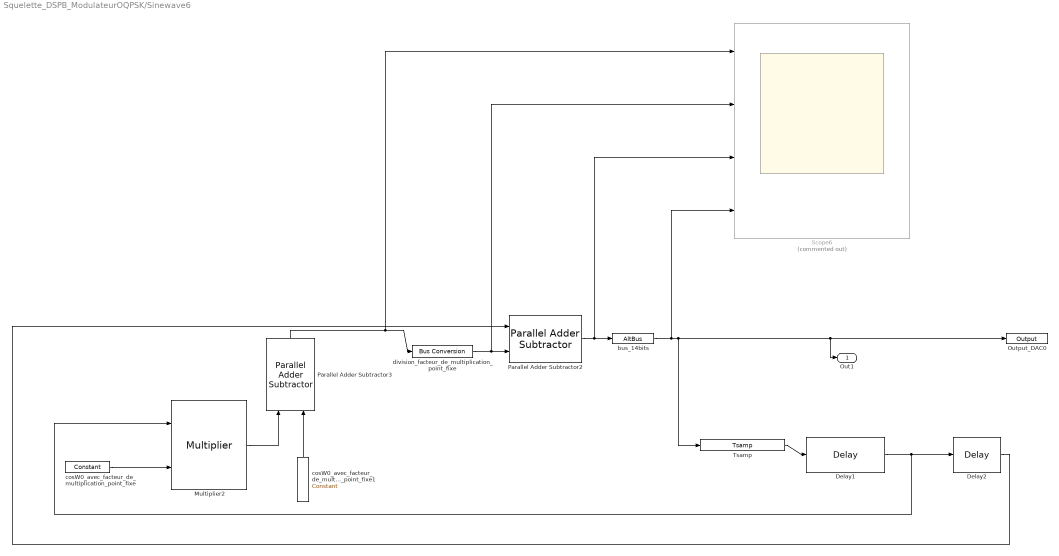
== system Squelette_DSPB_ModulateurOQPSK/Sinewave6 ==
  Delay1 : allblocks_alteradspbuilder2/Delay  pipeline=1  pipeline_display=1  ClockPhase=1  use_ena=off  use_sclr=off  allowFloatingPointOverride=on  logOutputs=off  logFile=U:\S6\Projet\Squelette_ModulateurOQPSK__ORIG\tb_Squelette_DSPB_ModulateurOQPSK\Squelette%5FDSPB%5FModulateurOQPSK_Sinewave6_Delay1.fixedpointlog  use_init=on  reset_value=0.031410759078128
  Delay2 : allblocks_alteradspbuilder2/Delay  pipeline=1  pipeline_display=1  ClockPhase=1  use_ena=off  use_sclr=off  allowFloatingPointOverride=on  logOutputs=off  logFile=U:\S6\Projet\Squelette_ModulateurOQPSK__ORIG\tb_Squelette_DSPB_ModulateurOQPSK\Squelette%5FDSPB%5FModulateurOQPSK_Sinewave6_Delay2.fixedpointlog  use_init=on  reset_value=0.062790519529314
  Multiplier2 : allblocks_alteradspbuilder2/Multiplier  BusType=Signed Fractional  bwl=8  bwr=20  pipeline=0  pipeline_display=0  allowFloatingPointOverride=on  logOutputs=off  logFile=U:\S6\Projet\Squelette_ModulateurOQPSK__ORIG\tb_Squelette_DSPB_ModulateurOQPSK\Squelette%5FDSPB%5FModulateurOQPSK_Sinewave6_Multiplier2.fixedpointlog  UseEqualInputWidth=off  bbwl=8  bbwr=20  FullResolution=on  OutputMsb=8  OutputLsb=0  OutputBwl=16  OutputBwr=16  UseDedicatedCircuitry=YES  use_ena=off  use_aclr=off
  Output_DAC0 : allblocks_alteradspbuilder2/Output  iofile=U:\S6\Projet\Squelette_ModulateurOQPSK__ORIG\tb_Squelette_DSPB_ModulateurOQPSK\Squelette%5FDSPB%5FModulateurOQPSK_Sinewave6_Output%5FDAC0.capture  BusType=Signed Integer  bwl=14  bwr=0  externalType=Inferred  PORTTYPE=Output  allowFloatingPointOverride=on  logOutputs=off
  Parallel Adder Subtractor2 : allblocks_alteradspbuilder2/Parallel Adder Subtractor  number_of_inputs=2  direction=-+  use_pipeline=off  pipeline_display=0  phase_selection=1  use_ena=off  use_aclr=off  allowFloatingPointOverride=on  logOutputs=off  logFile=U:\S6\Projet\Squelette_ModulateurOQPSK__ORIG\tb_Squelette_DSPB_ModulateurOQPSK\Squelette%5FDSPB%5FModulateurOQPSK_Sinewave6_Parallel+Adder+Subtractor2.fixedpointlog
  Parallel Adder Subtractor3 : allblocks_alteradspbuilder2/Parallel Adder Subtractor  number_of_inputs=2  direction=+  use_pipeline=off  pipeline_display=0  phase_selection=1  use_ena=off  use_aclr=off  allowFloatingPointOverride=on  logOutputs=off  logFile=U:\S6\Projet\Squelette_ModulateurOQPSK__ORIG\tb_Squelette_DSPB_ModulateurOQPSK\Squelette%5FDSPB%5FModulateurOQPSK_Sinewave6_Parallel+Adder+Subtractor3.fixedpointlog
  Scope6 : Scope  Commented=on  NumInputPorts=4
  Tsamp : allblocks_alteradspbuilder2/Tsamp  SpecifyClock=on  clock=Clock_100MHz
  bus_14bits : allblocks_alteradspbuilder2/AltBus  BusType=Signed Fractional  bwl=14  bwr=14  saturate=off  floatingPointInput=on  floatingPointOutput=on  logOutputs=off  logFile=U:\S6\Projet\Squelette_ModulateurOQPSK__ORIG\tb_Squelette_DSPB_ModulateurOQPSK\Squelette%5FDSPB%5FModulateurOQPSK_Sinewave6_bus%5F14bits.fixedpointlog
  cosW0_avec_facteur_de_multiplication_point_fixe : allblocks_alteradspbuilder2/Constant  mask_cst=1.999013120731463  BusType=Signed Fractional  bwl=19  bwr=19  roundMode=Truncate  satMode=Wrap  SpecifyClock=off  allowFloatingPointOverride=on  logOutputs=off  logFile=U:\S6\Projet\Squelette_ModulateurOQPSK__ORIG\tb_Squelette_DSPB_ModulateurOQPSK\Squelette%5FDSPB%5FModulateurOQPSK_Sinewave6_cosW0%5Favec%5Ffacteur%5Fde%5Fmultiplication%5Fpoint%5Ffixe.fixedpointlog
  cosW0_avec_facteur_de_multiplication_point_fixe1 : allblocks_alteradspbuilder2/Constant  mask_cst=2^-15  BusType=Signed Fractional  bwl=8  bwr=40  roundMode=Truncate  satMode=Wrap  SpecifyClock=off  allowFloatingPointOverride=on  logOutputs=off  logFile=U:\S6\Projet\Squelette_ModulateurOQPSK__ORIG\tb_Squelette_DSPB_ModulateurOQPSK\Squelette%5FDSPB%5FModulateurOQPSK_Sinewave6_cosW0%5Favec%5Ffacteur%5Fde%5Fmultiplication%5Fpoint%5Ffixe1.fixedpointlog
  division_facteur_de_multiplication_point_fixe : allblocks_alteradspbuilder2/Bus Conversion  BusType=Signed Fractional  ibwl=16  ibwr=40  bwl=8  bwr=20  bitToConnectToOutputLSB=16  round=off  saturate=off  pipeline_display=0
  Out1 : Outport
  wires:
  Parallel Adder Subtractor2/1 -> Scope6/3, bus_14bits/1
  Tsamp/1 -> Delay1/1
  cosW0_avec_facteur_de_multiplication_point_fixe1/1 -> Parallel Adder Subtractor3/2
  Multiplier2/1 -> Parallel Adder Subtractor3/1
  division_facteur_de_multiplication_point_fixe/1 -> Scope6/2, Parallel Adder Subtractor2/2
  Delay2/1 -> Parallel Adder Subtractor2/1
  Parallel Adder Subtractor3/1 -> Scope6/1, division_facteur_de_multiplication_point_fixe/1
  Delay1/1 -> Multiplier2/1, Delay2/1
  cosW0_avec_facteur_de_multiplication_point_fixe/1 -> Multiplier2/2
  bus_14bits/1 -> Scope6/4, Out1/1, Output_DAC0/1, Tsamp/1

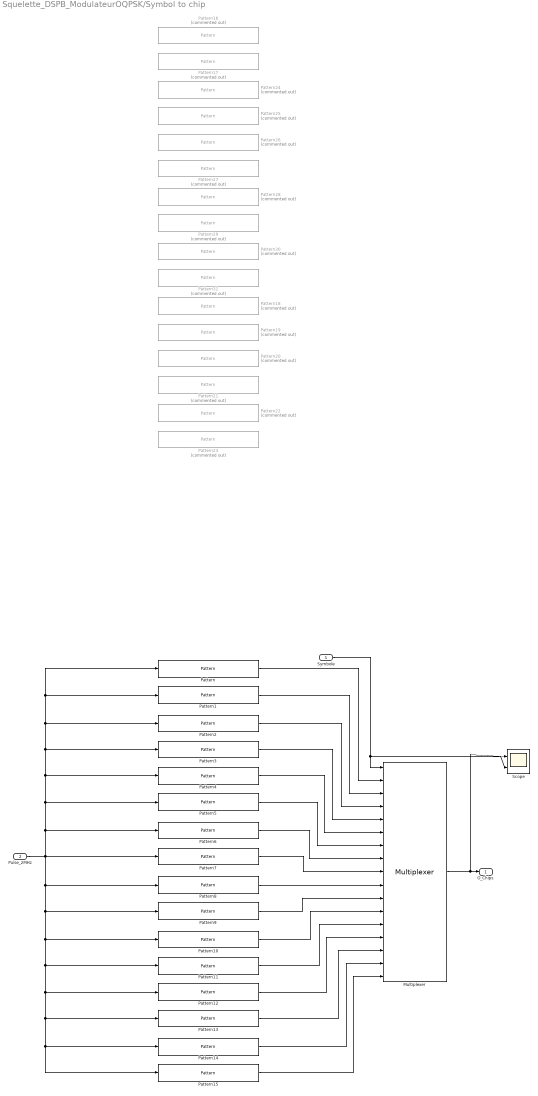
== system Squelette_DSPB_ModulateurOQPSK/Symbol to chip ==
  Symbole : Inport
  "Pulse_2MHz " : Inport  Port=2
  Multiplexer : allblocks_alteradspbuilder2/Multiplexer  numInputs=16  pipeline=0  oneHot=off  pipeline_display=0  use_ena=off  use_aclr=off  allowFloatingPointOverride=on  logOutputs=off  logFile=U:\S6\Projet\Squelette_ModulateurOQPSK__ORIG\tb_Squelette_DSPB_ModulateurOQPSK\Squelette%5FDSPB%5FModulateurOQPSK_Symbol+to+chip_Multiplexer.fixedpointlog
  Pattern : allblocks_alteradspbuilder2/Pattern  Sequence=11011001110000110101001000101110  SpecifyClock=off  use_ena=on  use_sclr=off
  Pattern1 : allblocks_alteradspbuilder2/Pattern  Sequence=11101101100111000011010100100010  SpecifyClock=off  use_ena=on  use_sclr=off
  Pattern10 : allblocks_alteradspbuilder2/Pattern  Sequence=01111011100011001001011000000111  SpecifyClock=off  use_ena=on  use_sclr=off
  Pattern11 : allblocks_alteradspbuilder2/Pattern  Sequence=01110111101110001100100101100000  SpecifyClock=off  use_ena=on  use_sclr=off
  Pattern12 : allblocks_alteradspbuilder2/Pattern  Sequence=00000111011110111000110010010110  SpecifyClock=off  use_ena=on  use_sclr=off
  Pattern13 : allblocks_alteradspbuilder2/Pattern  Sequence=01100000011101111011100011001001  SpecifyClock=off  use_ena=on  use_sclr=off
  Pattern14 : allblocks_alteradspbuilder2/Pattern  Sequence=10010110000001110111101110001100  SpecifyClock=off  use_ena=on  use_sclr=off
  Pattern15 : allblocks_alteradspbuilder2/Pattern  Sequence=1100100101100000111011110111000  SpecifyClock=off  use_ena=on  use_sclr=off
  Pattern16 : allblocks_alteradspbuilder2/Pattern  Commented=on  Sequence=01110100010010101100001110011011  SpecifyClock=off  use_ena=on  use_sclr=off
  Pattern17 : allblocks_alteradspbuilder2/Pattern  Commented=on  Sequence=01000100101011000011100110110111  SpecifyClock=off  use_ena=on  use_sclr=off
  Pattern18 : allblocks_alteradspbuilder2/Pattern  Commented=on  Sequence=11100000011010010011000111011110  SpecifyClock=off  use_ena=on  use_sclr=off
  Pattern19 : allblocks_alteradspbuilder2/Pattern  Commented=on  Sequence=00000110100100110001110111101110  SpecifyClock=off  use_ena=on  use_sclr=off
  Pattern2 : allblocks_alteradspbuilder2/Pattern  Sequence=00101110110110011100001101010010  SpecifyClock=off  use_ena=on  use_sclr=off
  Pattern20 : allblocks_alteradspbuilder2/Pattern  Commented=on  Sequence=01101001001100011101111011100000  SpecifyClock=off  use_ena=on  use_sclr=off
  Pattern21 : allblocks_alteradspbuilder2/Pattern  Commented=on  Sequence=10010011000111011110111000000110  SpecifyClock=off  use_ena=on  use_sclr=off
  Pattern22 : allblocks_alteradspbuilder2/Pattern  Commented=on  Sequence=00110001110111101110000001101001  SpecifyClock=off  use_ena=on  use_sclr=off
  Pattern23 : allblocks_alteradspbuilder2/Pattern  Commented=on  Sequence=00011101111011100000011010010011  SpecifyClock=off  use_ena=on  use_sclr=off
  Pattern24 : allblocks_alteradspbuilder2/Pattern  Commented=on  Sequence=01001010110000111001101101110100  SpecifyClock=off  use_ena=on  use_sclr=off
  Pattern25 : allblocks_alteradspbuilder2/Pattern  Commented=on  Sequence=10101100001110011011011101000100  SpecifyClock=off  use_ena=on  use_sclr=off
  Pattern26 : allblocks_alteradspbuilder2/Pattern  Commented=on  Sequence=11000011100110110111010001001010  SpecifyClock=off  use_ena=on  use_sclr=off
  Pattern27 : allblocks_alteradspbuilder2/Pattern  Commented=on  Sequence=00111001101101110100010010101100  SpecifyClock=off  use_ena=on  use_sclr=off
  Pattern28 : allblocks_alteradspbuilder2/Pattern  Commented=on  Sequence=10011011011101000100101011000011  SpecifyClock=off  use_ena=on  use_sclr=off
  Pattern29 : allblocks_alteradspbuilder2/Pattern  Commented=on  Sequence=10110111010001001010110000111001  SpecifyClock=off  use_ena=on  use_sclr=off
  Pattern3 : allblocks_alteradspbuilder2/Pattern  Sequence=00100010111011011001110000110101  SpecifyClock=off  use_ena=on  use_sclr=off
  Pattern30 : allblocks_alteradspbuilder2/Pattern  Commented=on  Sequence=11011110111000000110100100110001  SpecifyClock=off  use_ena=on  use_sclr=off
  Pattern31 : allblocks_alteradspbuilder2/Pattern  Commented=on  Sequence=11101110000001101001001100011101  SpecifyClock=off  use_ena=on  use_sclr=off
  Pattern4 : allblocks_alteradspbuilder2/Pattern  Sequence=01010010001011101101100111000011  SpecifyClock=off  use_ena=on  use_sclr=off
  Pattern5 : allblocks_alteradspbuilder2/Pattern  Sequence=00110101001000101110110110011100  SpecifyClock=off  use_ena=on  use_sclr=off
  Pattern6 : allblocks_alteradspbuilder2/Pattern  Sequence=11000011010100100010111011011001  SpecifyClock=off  use_ena=on  use_sclr=off
  Pattern7 : allblocks_alteradspbuilder2/Pattern  Sequence=10011100001101010010001011101101  SpecifyClock=off  use_ena=on  use_sclr=off
  Pattern8 : allblocks_alteradspbuilder2/Pattern  Sequence=10001100100101100000011101111011  SpecifyClock=off  use_ena=on  use_sclr=off
  Pattern9 : allblocks_alteradspbuilder2/Pattern  Sequence=10111000110010010110000001110111  SpecifyClock=off  use_ena=on  use_sclr=off
  Scope : Scope  NumInputPorts=2
  O_Chips : Outport
  wires:
  Pattern3/1 -> Multiplexer/5
  Pattern4/1 -> Multiplexer/6
  Pattern5/1 -> Multiplexer/7
  Pattern6/1 -> Multiplexer/8
  Pattern7/1 -> Multiplexer/9
  Pattern8/1 -> Multiplexer/10
  Pattern9/1 -> Multiplexer/11
  Pattern10/1 -> Multiplexer/12
  Pattern11/1 -> Multiplexer/13
  Pattern12/1 -> Multiplexer/14
  Pattern13/1 -> Multiplexer/15
  Pattern14/1 -> Multiplexer/16
  "Pulse_2MHz "/1 -> Pattern8/1, Pattern9/1, Pattern10/1, Pattern11/1, Pattern12/1, Pattern13/1, Pattern14/1, Pattern15/1, Pattern7/1, Pattern6/1, Pattern5/1, Pattern4/1, Pattern3/1, Pattern2/1, Pattern1/1, Pattern/1
  Pattern15/1 -> Multiplexer/17
  Pattern/1 -> Multiplexer/2
  Pattern1/1 -> Multiplexer/3
  Pattern2/1 -> Multiplexer/4
  Multiplexer/1 -> O_Chips/1, Scope/1
  Symbole/1 -> Scope/2, Multiplexer/1
